simulink model "Simulator_Case_5"  (R2024a)
settings: Solver=VariableStepAuto  StartTime=0.0  StopTime=2800  RelTol=1e-3
values from neighbouring files (symbols this model uses):
  Heading_Initial = -65*pi/180    (= -1.1344640138)    [Parametrization_Simulation_Case_5.m]
  Position_Initial_X = Waypoints_X(1)    [Parametrization_Simulation_Case_5.m]
  Position_Initial_Y = Waypoints_Y(1)    [Parametrization_Simulation_Case_5.m]
  Time_Period_Sampling = 0.1    [Parametrization_Simulation_Case_5.m]
undefined symbols (not defined in the file or in its folder): Area_Lateral_Projected_Wind, Damping_Factor_Waves, Density_Air, DiscIntNeverNeededParam, Gain_Proportional, Inertia_Moment, Length_Ship, Pulsation_Wave, Rudder_To_Heading_Discretized, Static_Gain_Nomoto, Structure_Wind_Coefficient, Time_Constant_Total, Time_Derivative, Time_Integral, Velocity_Ship_Mean, Wave_Transfer_Function_Discrete, Waypoints, Yaw_Control_Hydrodynamics_Derivative
libraries: simulink_extras x4, sensorgpslib x1
settings Model: Creator=gerar  LastModifiedBy=gerar

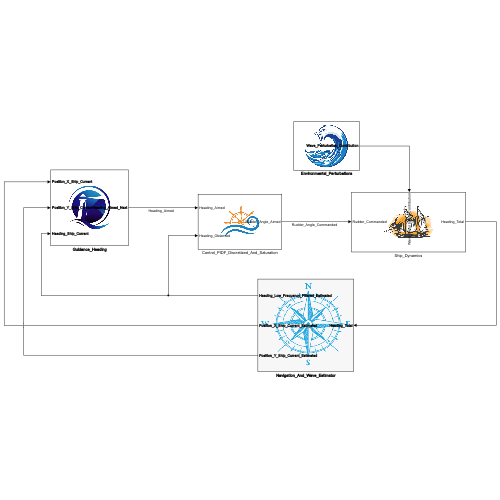
[thumbnail: Simulink's stored preview of the top-level diagram]
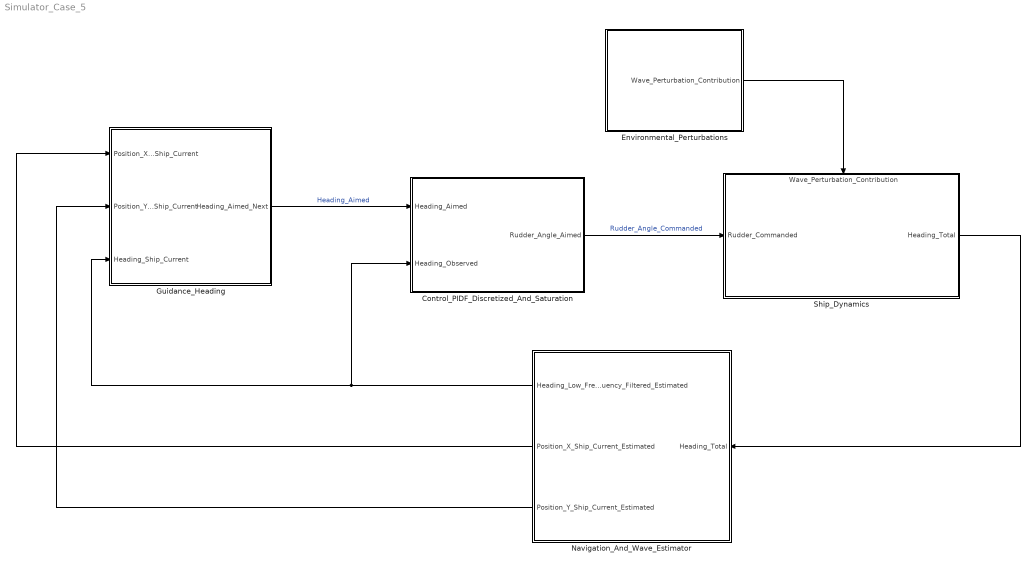
== system Simulator_Case_5 ==
  Control_PIDF_Discretized_And_Saturation : Subsystem
      mask Display: image('Rudder3.jpg');
  Environmental_Perturbations : Subsystem
      mask Display: image('Wave2.png');
  Guidance_Heading : Subsystem
      mask Display: image('phare4.jpg');
  Navigation_And_Wave_Estimator : Subsystem
      mask Display: image('compass4.png');
  Ship_Dynamics : Subsystem
      settings: PortSchema="{\"entries\":[{\"content\":{\"sides\":[{\"content\":{\"connectorIds\":[\"In1\"]},\"type\":\"ConnectorPlacement.EquallySpacedRectSide\",\"uuid\":\"1262d93f-9737-49c5-b1c8-13d3f825160d\"},{\"content\":{\"connectorIds\":[\"Out1\"],\"side\":\"RIGHT\"},\"type\":\"ConnectorPlacement.EquallySpacedRectSide\",\"uuid\":\"2783823e-17f0-4da0-9b4a-e84aa912eb5f\"},{\"content\":{\"connectorIds\":[\"In2\"],\"side\":\"TOP\"},\"type\":\"ConnectorPlacement.EquallySpacedRectSide\",\"uuid\":\"9227960a-c500-4bd1-9392-f2e1de824969\"}]},\"type\":\"ConnectorPlacement.EquallySpacedConnector\",\"uuid\":\"fe1a7a14-057d-49da-982c-994c0d128614\"}],\"packageUris\":[\"http://schema.mathworks.com/mf0/Connector/R2020b\"],\"version\":\"1.0\"}"
      mask Display: image('ship2.png');
  wires:
  Guidance_Heading/1(Heading_Aimed_Next) -> Control_PIDF_Discretized_And_Saturation/1(Heading_Aimed)  "Heading_Aimed"
  Navigation_And_Wave_Estimator/1(Heading_Low_Frequency_Filtered_Estimated) -> Control_PIDF_Discretized_And_Saturation/2(Heading_Observed), Guidance_Heading/3(Heading_Ship_Current)
  Control_PIDF_Discretized_And_Saturation/1(Rudder_Angle_Aimed) -> Ship_Dynamics/1(Rudder_Commanded)  "Rudder_Angle_Commanded"
  Environmental_Perturbations/1(Wave_Perturbation_Contribution) -> Ship_Dynamics/2(Wave_Perturbation_Contribution)
  Ship_Dynamics/1(Heading_Total) -> Navigation_And_Wave_Estimator/1(Heading_Total)
  Navigation_And_Wave_Estimator/3(Position_Y_Ship_Current_Estimated) -> Guidance_Heading/2(Position_Y_Ship_Current)
  Navigation_And_Wave_Estimator/2(Position_X_Ship_Current_Estimated) -> Guidance_Heading/1(Position_X_Ship_Current)

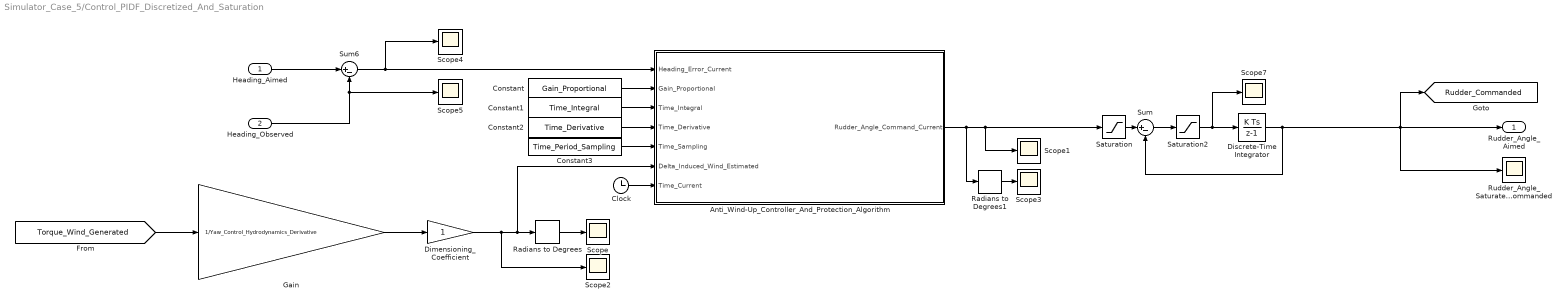
== system Simulator_Case_5/Control_PIDF_Discretized_And_Saturation ==
  Heading_Aimed : Inport
  Heading_Observed : Inport  Port=2
  Anti_Wind-Up_Controller_And_Protection_Algorithm : MATLAB Function  TreatAsAtomicUnit=on  SystemSampleTime=Time_Period_Sampling
  Clock : Clock
  Constant : Constant  Value=Gain_Proportional
  Constant1 : Constant  Value=Time_Integral
  Constant2 : Constant  Value=Time_Derivative
  Constant3 : Constant  Value=Time_Period_Sampling
  Dimensioning_Coefficient : Gain
  Discrete-Time Integrator : DiscreteIntegrator  SampleTime=Time_Period_Sampling  ICPrevOutput=DiscIntNeverNeededParam  ICPrevScaledInput=DiscIntNeverNeededParam
  Gain : Gain  Gain=1/Yaw_Control_Hydrodynamics_Derivative
  Radians to Degrees : simulink_extras/Transformations/Radians to Degrees
  Radians to Degrees1 : simulink_extras/Transformations/Radians to Degrees
  Rudder_Angle_Saturated_Commanded : Scope
  Saturation : Saturate  UpperLimit=35*(pi/180)  LowerLimit=-35*(pi/180)
  Saturation2 : Saturate  UpperLimit=15*(pi/180)  LowerLimit=-15*(pi/180)
  Scope{,1..5,7} (7 alike) : Scope
  Sum : Sum  Inputs=|+-
  Sum6 : Sum  Inputs=|+-
  Rudder_Angle_Aimed : Outport
  tag scope: Rudder_Commanded=global
  wires:
  Sum6/1 -> Scope4/1, Anti_Wind-Up_Controller_And_Protection_Algorithm/1(Heading_Error_Current)
  Heading_Aimed/1 -> Sum6/1
  Heading_Observed/1 -> Scope5/1, Sum6/2
  Constant/1 -> Anti_Wind-Up_Controller_And_Protection_Algorithm/2(Gain_Proportional)
  Constant1/1 -> Anti_Wind-Up_Controller_And_Protection_Algorithm/3(Time_Integral)
  Constant2/1 -> Anti_Wind-Up_Controller_And_Protection_Algorithm/4(Time_Derivative)
  Constant3/1 -> Anti_Wind-Up_Controller_And_Protection_Algorithm/5(Time_Sampling)
  [Torque_Wind_Generated] -> Gain/1
  Gain/1 -> Dimensioning_Coefficient/1
  Radians to Degrees/1 -> Scope/1
  Radians to Degrees1/1 -> Scope3/1
  Anti_Wind-Up_Controller_And_Protection_Algorithm/1(Rudder_Angle_Command_Current) -> Radians to Degrees1/1, Saturation/1, Scope1/1
  Dimensioning_Coefficient/1 -> Anti_Wind-Up_Controller_And_Protection_Algorithm/6(Delta_Induced_Wind_Estimated), Radians to Degrees/1, Scope2/1
  Clock/1 -> Anti_Wind-Up_Controller_And_Protection_Algorithm/7(Time_Current)
  Saturation2/1 -> Scope7/1, Discrete-Time Integrator/1
  Saturation/1 -> Sum/1
  Sum/1 -> Saturation2/1
  Discrete-Time Integrator/1 -> Sum/2, Rudder_Angle_Saturated_Commanded/1, [Rudder_Commanded], Rudder_Angle_Aimed/1

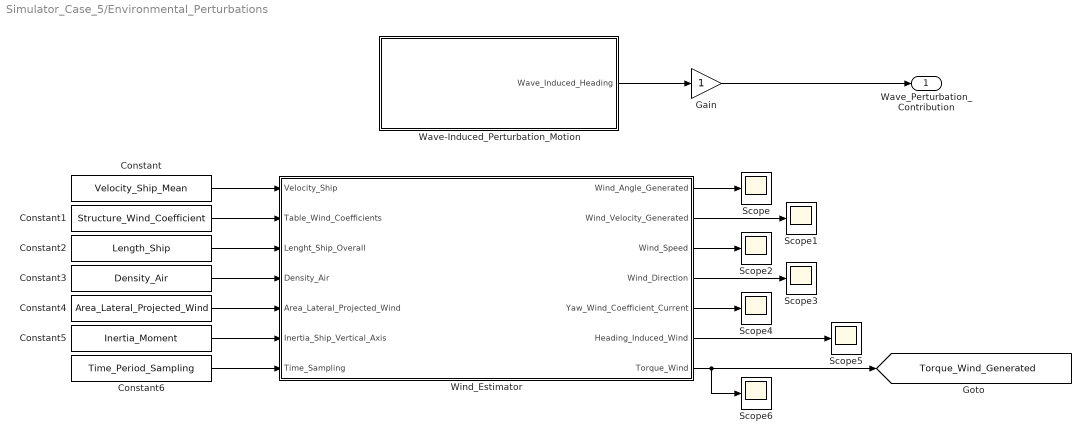
== system Simulator_Case_5/Environmental_Perturbations ==
  Constant : Constant  Value=Velocity_Ship_Mean
  Constant1 : Constant  Value=Structure_Wind_Coefficient
  Constant2 : Constant  Value=Length_Ship
  Constant3 : Constant  Value=Density_Air
  Constant4 : Constant  Value=Area_Lateral_Projected_Wind
  Constant5 : Constant  Value=Inertia_Moment
  Constant6 : Constant  Value=Time_Period_Sampling
  Gain : Gain
  Scope{,1..6} (7 alike) : Scope
  Wave-Induced_Perturbation_Motion : Subsystem
  Wind_Estimator : MATLAB Function  TreatAsAtomicUnit=on  SystemSampleTime=Time_Period_Sampling
  Wave_Perturbation_Contribution : Outport
  tag scope: Torque_Wind_Generated=global
  wires:
  Wave-Induced_Perturbation_Motion/1(Wave_Induced_Heading) -> Gain/1
  Constant/1 -> Wind_Estimator/1(Velocity_Ship)
  Constant1/1 -> Wind_Estimator/2(Table_Wind_Coefficients)
  Constant2/1 -> Wind_Estimator/3(Lenght_Ship_Overall)
  Constant3/1 -> Wind_Estimator/4(Density_Air)
  Constant4/1 -> Wind_Estimator/5(Area_Lateral_Projected_Wind)
  Constant5/1 -> Wind_Estimator/6(Inertia_Ship_Vertical_Axis)
  Wind_Estimator/1(Wind_Angle_Generated) -> Scope/1
  Wind_Estimator/2(Wind_Velocity_Generated) -> Scope1/1
  Wind_Estimator/3(Wind_Speed) -> Scope2/1
  Wind_Estimator/4(Wind_Direction) -> Scope3/1
  Wind_Estimator/5(Yaw_Wind_Coefficient_Current) -> Scope4/1
  Wind_Estimator/6(Heading_Induced_Wind) -> Scope5/1
  Wind_Estimator/7(Torque_Wind) -> Scope6/1, [Torque_Wind_Generated]
  Constant6/1 -> Wind_Estimator/7(Time_Sampling)
  Gain/1 -> Wave_Perturbation_Contribution/1

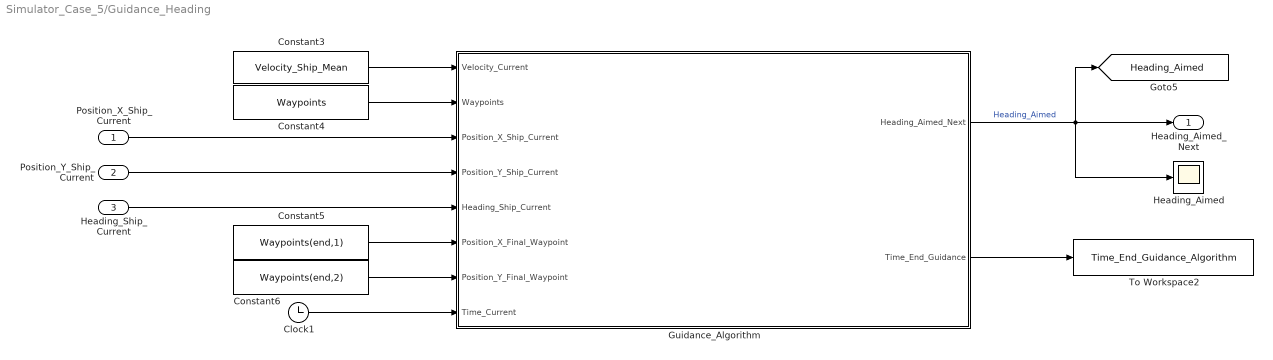
== system Simulator_Case_5/Guidance_Heading ==
  Position_X_Ship_Current : Inport
  Position_Y_Ship_Current : Inport  Port=2
  Heading_Ship_Current : Inport  Port=3
  Clock1 : Clock
  Constant3 : Constant  Value=Velocity_Ship_Mean
  Constant4 : Constant  Value=Waypoints
  Constant5 : Constant  Value=Waypoints(end,1)
  Constant6 : Constant  Value=Waypoints(end,2)
  Guidance_Algorithm : MATLAB Function  TreatAsAtomicUnit=on  SystemSampleTime=20
  Heading_Aimed : Scope
  To Workspace2 : ToWorkspace  VariableName=Time_End_Guidance_Algorithm  SaveFormat=Timeseries  SampleTime=-1
  Heading_Aimed_Next : Outport
  tag scope: Heading_Aimed=global
  wires:
  Constant5/1 -> Guidance_Algorithm/6(Position_X_Final_Waypoint)
  Guidance_Algorithm/2(Time_End_Guidance) -> To Workspace2/1
  Constant3/1 -> Guidance_Algorithm/1(Velocity_Current)
  Position_Y_Ship_Current/1 -> Guidance_Algorithm/4(Position_Y_Ship_Current)
  Constant4/1 -> Guidance_Algorithm/2(Waypoints)
  Clock1/1 -> Guidance_Algorithm/8(Time_Current)
  Constant6/1 -> Guidance_Algorithm/7(Position_Y_Final_Waypoint)
  Position_X_Ship_Current/1 -> Guidance_Algorithm/3(Position_X_Ship_Current)
  Heading_Ship_Current/1 -> Guidance_Algorithm/5(Heading_Ship_Current)
  Guidance_Algorithm/1(Heading_Aimed_Next) -> Heading_Aimed/1, Heading_Aimed_Next/1, [Heading_Aimed]  "Heading_Aimed"

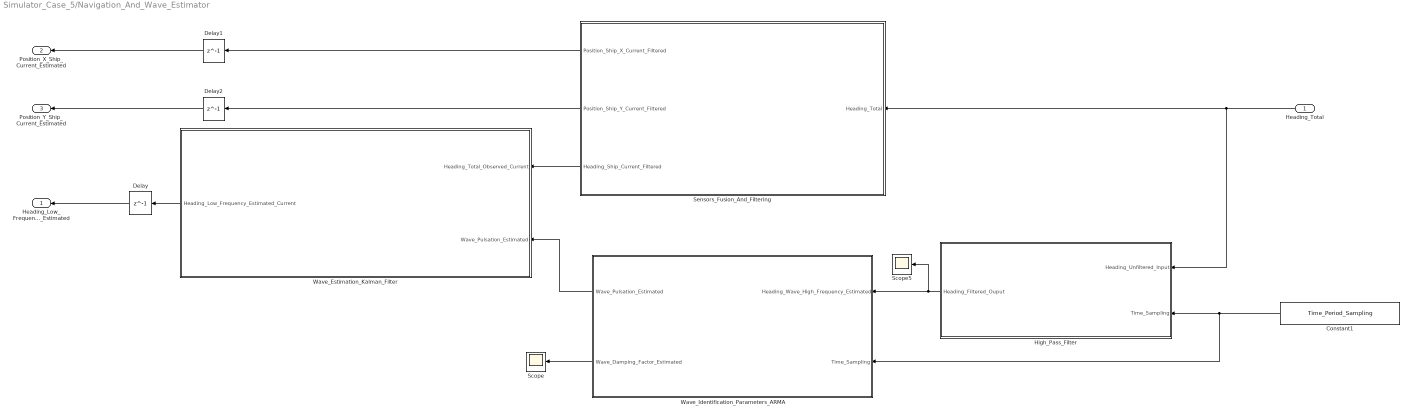
== system Simulator_Case_5/Navigation_And_Wave_Estimator ==
  Heading_Total : Inport
  Constant1 : Constant  Value=Time_Period_Sampling
  Delay : Delay  DelayLength=1  InputProcessing=Columns as channels (frame based)  SampleTime=0.1
  Delay1 : Delay  DelayLength=1  InputProcessing=Columns as channels (frame based)  SampleTime=0.1
  Delay2 : Delay  DelayLength=1  InputProcessing=Columns as channels (frame based)  SampleTime=0.1
  High_Pass_Filter : MATLAB Function  TreatAsAtomicUnit=on  SystemSampleTime=Time_Period_Sampling
  Scope : Scope
  Scope5 : Scope
  Sensors_Fusion_And_Filtering : Subsystem
  Wave_Estimation_Kalman_Filter : Subsystem
  Wave_Identification_Parameters_ARMA : MATLAB Function  TreatAsAtomicUnit=on  SystemSampleTime=Time_Period_Sampling
  Heading_Low_Frequency_Filtered_Estimated : Outport
  Position_X_Ship_Current_Estimated : Outport  Port=2
  Position_Y_Ship_Current_Estimated : Outport  Port=3
  wires:
  Delay/1 -> Heading_Low_Frequency_Filtered_Estimated/1
  Delay1/1 -> Position_X_Ship_Current_Estimated/1
  Delay2/1 -> Position_Y_Ship_Current_Estimated/1
  Sensors_Fusion_And_Filtering/1(Position_Ship_X_Current_Filtered) -> Delay1/1
  Sensors_Fusion_And_Filtering/2(Position_Ship_Y_Current_Filtered) -> Delay2/1
  Sensors_Fusion_And_Filtering/3(Heading_Ship_Current_Filtered) -> Wave_Estimation_Kalman_Filter/1(Heading_Total_Observed_Current)
  Wave_Estimation_Kalman_Filter/1(Heading_Low_Frequency_Estimated_Current) -> Delay/1
  High_Pass_Filter/1(Heading_Filtered_Ouput) -> Scope5/1, Wave_Identification_Parameters_ARMA/1(Heading_Wave_High_Frequency_Estimated)
  Constant1/1 -> Wave_Identification_Parameters_ARMA/2(Time_Sampling), High_Pass_Filter/2(Time_Sampling)
  Wave_Identification_Parameters_ARMA/2(Wave_Damping_Factor_Estimated) -> Scope/1
  Wave_Identification_Parameters_ARMA/1(Wave_Pulsation_Estimated) -> Wave_Estimation_Kalman_Filter/2(Wave_Pulsation_Estimated)
  Heading_Total/1 -> High_Pass_Filter/1(Heading_Unfiltered_Input), Sensors_Fusion_And_Filtering/1(Heading_Total)

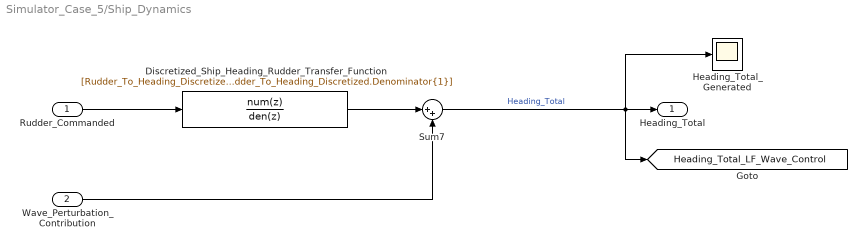
== system Simulator_Case_5/Ship_Dynamics ==
  Rudder_Commanded : Inport
  Wave_Perturbation_Contribution : Inport  Port=2
  Discretized_Ship_Heading_Rudder_Transfer_Function : DiscreteTransferFcn  Numerator=[Rudder_To_Heading_Discretized.Numerator{1}]  Denominator=[Rudder_To_Heading_Discretized.Denominator{1}]  InitialStates=Heading_Initial
  Heading_Total_Generated : Scope
  Sum7 : Sum  Inputs=|++
  Heading_Total : Outport
  tag scope: Heading_Total_LF_Wave_Control=global
  wires:
  Discretized_Ship_Heading_Rudder_Transfer_Function/1 -> Sum7/1
  Wave_Perturbation_Contribution/1 -> Sum7/2
  Rudder_Commanded/1 -> Discretized_Ship_Heading_Rudder_Transfer_Function/1
  Sum7/1 -> [Heading_Total_LF_Wave_Control], Heading_Total/1, Heading_Total_Generated/1  "Heading_Total"

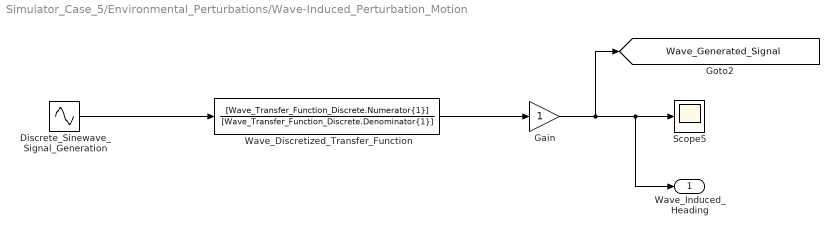
== system Simulator_Case_5/Environmental_Perturbations/Wave-Induced_Perturbation_Motion ==
  Discrete_Sinewave_Signal_Generation : Sin  Amplitude=5*(pi/180)  Frequency=Pulsation_Wave  SampleTime=Time_Period_Sampling
  Gain : Gain
  Scope5 : Scope
  Wave_Discretized_Transfer_Function : DiscreteTransferFcn  Numerator=[Wave_Transfer_Function_Discrete.Numerator{1}]  Denominator=[Wave_Transfer_Function_Discrete.Denominator{1}]
  Wave_Induced_Heading : Outport
  tag scope: Wave_Generated_Signal=global
  wires:
  Gain/1 -> Wave_Induced_Heading/1, Scope5/1, [Wave_Generated_Signal]
  Discrete_Sinewave_Signal_Generation/1 -> Wave_Discretized_Transfer_Function/1
  Wave_Discretized_Transfer_Function/1 -> Gain/1

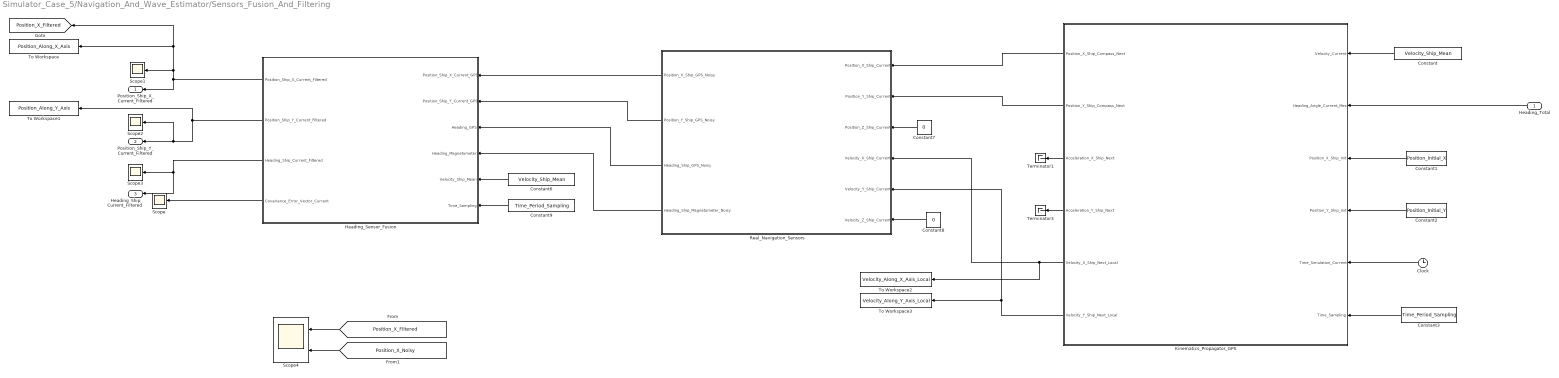
== system Simulator_Case_5/Navigation_And_Wave_Estimator/Sensors_Fusion_And_Filtering ==
  Heading_Total : Inport
  Clock : Clock
  Constant : Constant  Value=Velocity_Ship_Mean
  Constant1 : Constant  Value=Position_Initial_X
  Constant2 : Constant  Value=Position_Initial_Y
  Constant3 : Constant  Value=Time_Period_Sampling
  Constant6 : Constant  Value=Velocity_Ship_Mean
  Constant7 : Constant  Value=0
  Constant8 : Constant  Value=0
  Constant9 : Constant  Value=Time_Period_Sampling
  Heading_Sensor_Fusion : MATLAB Function  TreatAsAtomicUnit=on  SystemSampleTime=Time_Period_Sampling
  Kinematics_Propagator_GPS : MATLAB Function  TreatAsAtomicUnit=on  SystemSampleTime=Time_Period_Sampling
  Real_Navigation_Sensors : Subsystem
  Scope{,1..3} (4 alike) : Scope
  Scope4 : Scope  NumInputPorts=2
  Terminator1 : Terminator
  Terminator3 : Terminator
  To Workspace : ToWorkspace  VariableName=Position_Along_X_Axis  SaveFormat=Timeseries  SampleTime=Time_Period_Sampling
  To Workspace1 : ToWorkspace  VariableName=Position_Along_Y_Axis  SaveFormat=Timeseries  SampleTime=Time_Period_Sampling
  To Workspace2 : ToWorkspace  VariableName=Velocity_Along_X_Axis_Local  SaveFormat=Timeseries  SampleTime=Time_Period_Sampling
  To Workspace3 : ToWorkspace  VariableName=Velocity_Along_Y_Axis_Local  SaveFormat=Timeseries  SampleTime=Time_Period_Sampling
  Position_Ship_X_Current_Filtered : Outport
  Position_Ship_Y_Current_Filtered : Outport  Port=2
  Heading_Ship_Current_Filtered : Outport  Port=3
  tag scope: Position_X_Filtered=global
  wires:
  Real_Navigation_Sensors/1(Position_X_Ship_GPS_Noisy) -> Heading_Sensor_Fusion/1(Position_Ship_X_Current_GPS)
  Real_Navigation_Sensors/3(Heading_Ship_GPS_Noisy) -> Heading_Sensor_Fusion/3(Heading_GPS)
  Constant6/1 -> Heading_Sensor_Fusion/5(Velocity_Ship_Mean)
  Real_Navigation_Sensors/4(Heading_Ship_Magnetometer_Noisy) -> Heading_Sensor_Fusion/4(Heading_Magnetometer)
  Real_Navigation_Sensors/2(Position_Y_Ship_GPS_Noisy) -> Heading_Sensor_Fusion/2(Position_Ship_Y_Current_GPS)
  Constant2/1 -> Kinematics_Propagator_GPS/4(Position_Y_Ship_Init)
  Heading_Total/1 -> Kinematics_Propagator_GPS/2(Heading_Angle_Current_Mes)
  Clock/1 -> Kinematics_Propagator_GPS/5(Time_Simulation_Current)
  Constant1/1 -> Kinematics_Propagator_GPS/3(Position_X_Ship_Init)
  Constant/1 -> Kinematics_Propagator_GPS/1(Velocity_Current)
  Constant3/1 -> Kinematics_Propagator_GPS/6(Time_Sampling)
  Kinematics_Propagator_GPS/1(Position_X_Ship_Compass_Next) -> Real_Navigation_Sensors/1(Position_X_Ship_Current)
  Kinematics_Propagator_GPS/2(Position_Y_Ship_Compass_Next) -> Real_Navigation_Sensors/2(Position_Y_Ship_Current)
  Kinematics_Propagator_GPS/5(Velocity_X_Ship_Next_Local) -> Real_Navigation_Sensors/4(Velocity_X_Ship_Current), To Workspace2/1
  Kinematics_Propagator_GPS/6(Velocity_Y_Ship_Next_Local) -> To Workspace3/1, Real_Navigation_Sensors/5(Velocity_Y_Ship_Current)
  Constant7/1 -> Real_Navigation_Sensors/3(Position_Z_Ship_Current)
  Constant8/1 -> Real_Navigation_Sensors/6(Velocity_Z_Ship_Current)
  Constant9/1 -> Heading_Sensor_Fusion/6(Time_Sampling)
  Heading_Sensor_Fusion/1(Position_Ship_X_Current_Filtered) -> Position_Ship_X_Current_Filtered/1, [Position_X_Filtered], To Workspace/1, Scope1/1
  Heading_Sensor_Fusion/2(Position_Ship_Y_Current_Filtered) -> Scope2/1, Position_Ship_Y_Current_Filtered/1, To Workspace1/1
  Heading_Sensor_Fusion/3(Heading_Ship_Current_Filtered) -> Heading_Ship_Current_Filtered/1, Scope3/1
  Heading_Sensor_Fusion/4(Covariance_Error_Vector_Current) -> Scope/1
  Kinematics_Propagator_GPS/3(Acceleration_X_Ship_Next) -> Terminator1/1
  Kinematics_Propagator_GPS/4(Acceleration_Y_Ship_Next) -> Terminator3/1
  [Position_X_Filtered] -> Scope4/1
  [Position_X_Noisy] -> Scope4/2

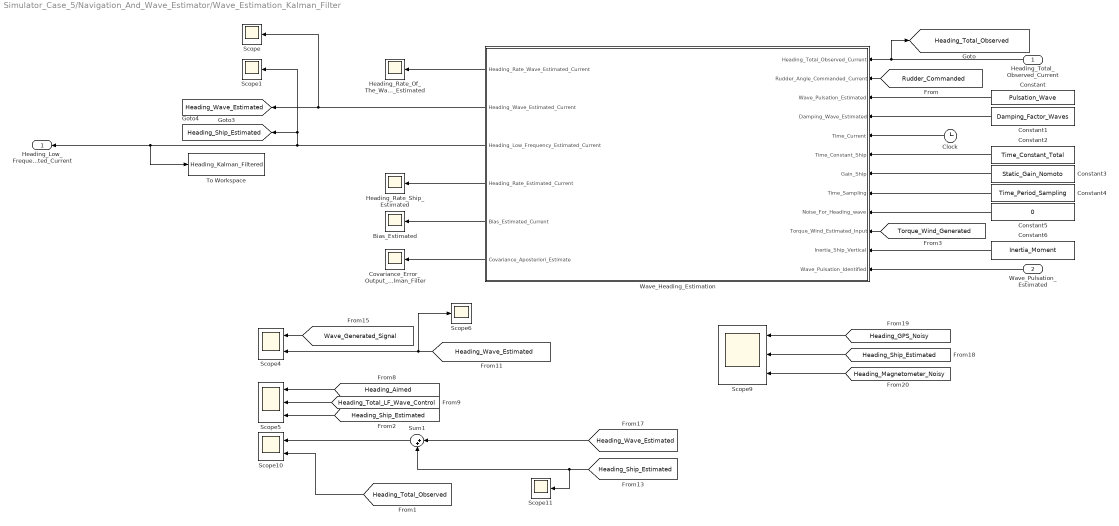
== system Simulator_Case_5/Navigation_And_Wave_Estimator/Wave_Estimation_Kalman_Filter ==
  Heading_Total_Observed_Current : Inport
  Wave_Pulsation_Estimated : Inport  Port=2
  Bias_Estimated : Scope
  Clock : Clock
  Constant : Constant  Value=Pulsation_Wave  SampleTime=Time_Period_Sampling
  Constant1 : Constant  Value=Damping_Factor_Waves  SampleTime=Time_Period_Sampling
  Constant2 : Constant  Value=Time_Constant_Total  SampleTime=Time_Period_Sampling
  Constant3 : Constant  Value=Static_Gain_Nomoto  SampleTime=Time_Period_Sampling
  Constant4 : Constant  Value=Time_Period_Sampling  SampleTime=Time_Period_Sampling
  Constant5 : Constant  Value=0
  Constant6 : Constant  Value=Inertia_Moment
  Covariance_Error_Output_Kalman_Filter : Scope
  Heading_Rate_Of_The_Waves_Estimated : Scope
  Heading_Rate_Ship_Estimated : Scope
  Scope{,1,6,11} (4 alike) : Scope
  Scope10 : Scope  NumInputPorts=2
  Scope4 : Scope  NumInputPorts=2
  Scope5 : Scope  NumInputPorts=3
  Scope9 : Scope  NumInputPorts=3
  Sum1 : Sum  Inputs=|++
  To Workspace : ToWorkspace  VariableName=Heading_Kalman_Filtered  SaveFormat=Timeseries  SampleTime=Time_Period_Sampling
  Wave_Heading_Estimation : MATLAB Function  TreatAsAtomicUnit=on  SystemSampleTime=Time_Period_Sampling
  Heading_Low_Frequency_Estimated_Current : Outport
  tag scope: Heading_Ship_Estimated=global, Heading_Total_Observed=global, Heading_Wave_Estimated=global
  wires:
  Wave_Heading_Estimation/3(Heading_Low_Frequency_Estimated_Current) -> Scope1/1, [Heading_Ship_Estimated], Heading_Low_Frequency_Estimated_Current/1, To Workspace/1
  Heading_Total_Observed_Current/1 -> [Heading_Total_Observed], Wave_Heading_Estimation/1(Heading_Total_Observed_Current)
  [Rudder_Commanded] -> Wave_Heading_Estimation/2(Rudder_Angle_Commanded_Current)
  Constant/1 -> Wave_Heading_Estimation/3(Wave_Pulsation_Estimated)
  Constant1/1 -> Wave_Heading_Estimation/4(Damping_Wave_Estimated)
  Clock/1 -> Wave_Heading_Estimation/5(Time_Current)
  Constant2/1 -> Wave_Heading_Estimation/6(Time_Constant_Ship)
  Constant3/1 -> Wave_Heading_Estimation/7(Gain_Ship)
  Constant4/1 -> Wave_Heading_Estimation/8(Time_Sampling)
  Constant5/1 -> Wave_Heading_Estimation/9(Noise_For_Heading_wave)
  Wave_Heading_Estimation/1(Heading_Rate_Wave_Estimated_Current) -> Heading_Rate_Of_The_Waves_Estimated/1
  Wave_Heading_Estimation/2(Heading_Wave_Estimated_Current) -> Scope/1, [Heading_Wave_Estimated]
  Wave_Heading_Estimation/5(Bias_Estimated_Current) -> Bias_Estimated/1
  Wave_Heading_Estimation/4(Heading_Rate_Estimated_Current) -> Heading_Rate_Ship_Estimated/1
  Wave_Heading_Estimation/6(Covariance_Aposteriori_Estimate) -> Covariance_Error_Output_Kalman_Filter/1
  [Heading_Aimed] -> Scope5/1
  [Wave_Generated_Signal] -> Scope4/1
  [Heading_Ship_Estimated] -> Scope9/2
  [Heading_Magnetometer_Noisy] -> Scope9/3
  [Heading_Ship_Estimated] -> Scope11/1, Sum1/2
  [Heading_GPS_Noisy] -> Scope9/1
  [Heading_Wave_Estimated] -> Sum1/1
  Sum1/1 -> Scope10/1
  [Heading_Total_LF_Wave_Control] -> Scope5/2
  [Heading_Ship_Estimated] -> Scope5/3
  [Heading_Wave_Estimated] -> Scope6/1, Scope4/2
  [Heading_Total_Observed] -> Scope10/2
  Constant6/1 -> Wave_Heading_Estimation/11(Inertia_Ship_Vertical)
  [Torque_Wind_Generated] -> Wave_Heading_Estimation/10(Torque_Wind_Estimated_Input)
  Wave_Pulsation_Estimated/1 -> Wave_Heading_Estimation/12(Wave_Pulsation_Identified)

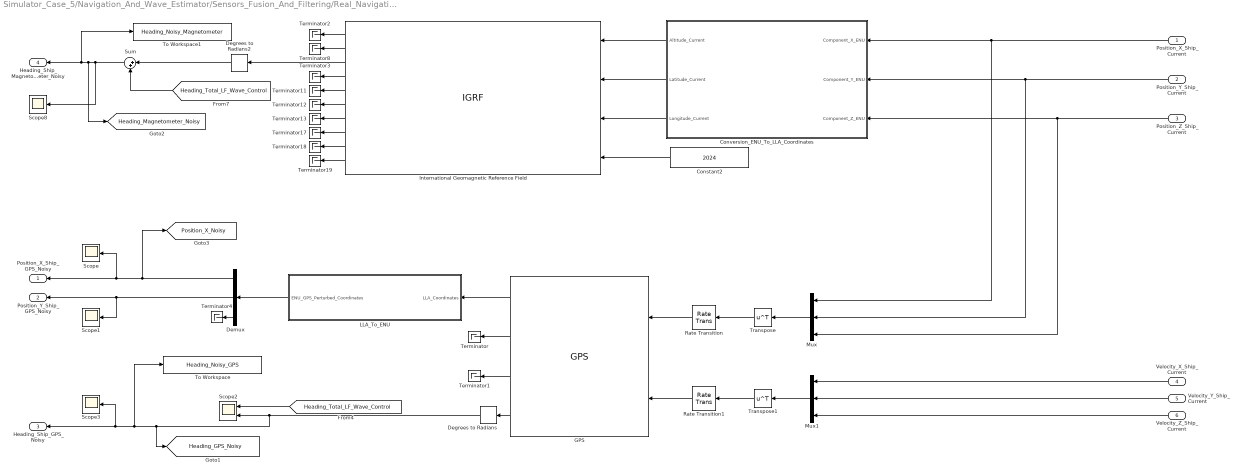
== system Simulator_Case_5/Navigation_And_Wave_Estimator/Sensors_Fusion_And_Filtering/Real_Navigation_Sensors ==
  Position_X_Ship_Current : Inport
  Position_Y_Ship_Current : Inport  Port=2
  Position_Z_Ship_Current : Inport  Port=3
  Velocity_X_Ship_Current : Inport  Port=4
  Velocity_Y_Ship_Current : Inport  Port=5
  Velocity_Z_Ship_Current : Inport  Port=6
  Constant2 : Constant  Value=2024
  Conversion_ENU_To_LLA_Coordinates : MATLAB Function  TreatAsAtomicUnit=on  SystemSampleTime=Time_Period_Sampling
  Degrees to Radians : simulink_extras/Transformations/Degrees to Radians
  Degrees to Radians2 : simulink_extras/Transformations/Degrees to Radians
  Demux : Demux  Outputs=3
  GPS : sensorgpslib/GPS  DispRefFrame=ENU  PositionInputFormat=Local  ReferenceLocation=[43.059023, 3.002915 ,0]  HorizontalPositionAccuracy=2  VerticalPositionAccuracy=2  VelocityAccuracy=0.1  DecayFactor=0.999  SeedDouble=67  SimulateUsing=Interpreted execution
  International Geomagnetic Reference Field : IGRF  month=January  day=1  year=2020
      settings: AttributesFormatString=%<generation>
  LLA_To_ENU : MATLAB Function  TreatAsAtomicUnit=on  SystemSampleTime=Time_Period_Sampling
  Mux : Mux  Inputs=3
  Mux1 : Mux  Inputs=3
  Rate Transition : RateTransition  OutPortSampleTime=Time_Period_Sampling
  Rate Transition1 : RateTransition  OutPortSampleTime=Time_Period_Sampling
  Scope{,1,3,8} (4 alike) : Scope
  Scope2 : Scope  NumInputPorts=2
  Sum : Sum  Inputs=|++
  Terminator{,1..4,8,11..13,17..19} (12 alike) : Terminator
  To Workspace : ToWorkspace  VariableName=Heading_Noisy_GPS  SaveFormat=Timeseries  SampleTime=Time_Period_Sampling
  To Workspace1 : ToWorkspace  VariableName=Heading_Noisy_Magnetometer  SaveFormat=Timeseries  SampleTime=Time_Period_Sampling
  Transpose : Math  Operator=transpose
  Transpose1 : Math  Operator=transpose
  Position_X_Ship_GPS_Noisy : Outport
  Position_Y_Ship_GPS_Noisy : Outport  Port=2
  Heading_Ship_GPS_Noisy : Outport  Port=3
  Heading_Ship_Magnetometer_Noisy : Outport  Port=4
  tag scope: Heading_GPS_Noisy=global, Heading_Magnetometer_Noisy=global, Position_X_Noisy=global
  wires:
  [Heading_Total_LF_Wave_Control] -> Scope2/1
  International Geomagnetic Reference Field/1 -> Terminator2/1
  Position_Y_Ship_Current/1 -> Mux/2, Conversion_ENU_To_LLA_Coordinates/2(Component_Y_ENU)
  GPS/3 -> Terminator1/1
  International Geomagnetic Reference Field/6 -> Terminator12/1
  International Geomagnetic Reference Field/10 -> Terminator19/1
  Demux/2 -> Position_Y_Ship_GPS_Noisy/1, Scope1/1
  International Geomagnetic Reference Field/5 -> Terminator11/1
  Degrees to Radians/1 -> [Heading_GPS_Noisy], To Workspace/1, Heading_Ship_GPS_Noisy/1, Scope3/1, Scope2/2
  Velocity_Y_Ship_Current/1 -> Mux1/2
  Conversion_ENU_To_LLA_Coordinates/1(Altitude_Current) -> International Geomagnetic Reference Field/1
  Demux/3 -> Terminator4/1
  Degrees to Radians2/1 -> Sum/1
  Mux/1 -> Transpose/1
  Position_X_Ship_Current/1 -> Mux/1, Conversion_ENU_To_LLA_Coordinates/1(Component_X_ENU)
  [Heading_Total_LF_Wave_Control] -> Sum/2
  Constant2/1 -> International Geomagnetic Reference Field/4
  GPS/4 -> Degrees to Radians/1
  GPS/2 -> Terminator/1
  International Geomagnetic Reference Field/4 -> Terminator3/1
  Rate Transition1/1 -> GPS/2
  Demux/1 -> [Position_X_Noisy], Position_X_Ship_GPS_Noisy/1, Scope/1
  International Geomagnetic Reference Field/8 -> Terminator17/1
  International Geomagnetic Reference Field/2 -> Terminator8/1
  Transpose1/1 -> Rate Transition1/1
  Conversion_ENU_To_LLA_Coordinates/2(Latitude_Current) -> International Geomagnetic Reference Field/2
  Transpose/1 -> Rate Transition/1
  Rate Transition/1 -> GPS/1
  Position_Z_Ship_Current/1 -> Mux/3, Conversion_ENU_To_LLA_Coordinates/3(Component_Z_ENU)
  LLA_To_ENU/1(ENU_GPS_Perturbed_Coordinates) -> Demux/1
  Mux1/1 -> Transpose1/1
  International Geomagnetic Reference Field/3 -> Degrees to Radians2/1
  GPS/1 -> LLA_To_ENU/1(LLA_Coordinates)
  Conversion_ENU_To_LLA_Coordinates/3(Longitude_Current) -> International Geomagnetic Reference Field/3
  International Geomagnetic Reference Field/7 -> Terminator13/1
  International Geomagnetic Reference Field/9 -> Terminator18/1
  Velocity_Z_Ship_Current/1 -> Mux1/3
  Velocity_X_Ship_Current/1 -> Mux1/1
  Sum/1 -> To Workspace1/1, Heading_Ship_Magnetometer_Noisy/1, [Heading_Magnetometer_Noisy], Scope8/1

== matlab function Simulator_Case_5/Navigation_And_Wave_Estimator/Sensors_Fusion_And_Filtering/Heading_Sensor_Fusion ==
  settings: updateMethod=DISCRETE
  data: Position_Ship_X_Current_GPS input; Position_Ship_Y_Current_GPS input; Heading_GPS input; Heading_Magnetometer input; Position_Ship_X_Current_Filtered output; Position_Ship_Y_Current_Filtered output; Heading_Ship_Current_Filtered output; Covariance_Error_Vector_Current output; Velocity_Ship_Mean input; Time_Sampling input
function [Position_Ship_X_Current_Filtered,...
          Position_Ship_Y_Current_Filtered,...
          Heading_Ship_Current_Filtered,...
          Covariance_Error_Vector_Current]  = Navigation_Kalman_Sensor_Fusion(Position_Ship_X_Current_GPS,...
                                                                              Position_Ship_Y_Current_GPS,...
                                                                              Heading_GPS,...
                                                                              Heading_Magnetometer,...
                                                                              Velocity_Ship_Mean,...
                                                                              Time_Sampling)

% Online Sensor Fusion and Filtering algorithm:
[Position_Ship_X_Current_Filtered,...
 Position_Ship_Y_Current_Filtered,...
 Heading_Ship_Current_Filtered,...
 Covariance_Error_Vector_Current] = Navigation_Kalman_Fusion_Positions_Heading(Position_Ship_X_Current_GPS,...
                                                                               Position_Ship_Y_Current_GPS,...
                                                                               Heading_GPS,...
                                                                               Heading_Magnetometer,...
                                                                               Velocity_Ship_Mean,...
                                                                               Time_Sampling);

end

== matlab function Simulator_Case_5/Navigation_And_Wave_Estimator/Sensors_Fusion_And_Filtering/Real_Navigation_Sensors/LLA_To_ENU ==
  data: LLA_Coordinates input; ENU_GPS_Perturbed_Coordinates output
function ENU_GPS_Perturbed_Coordinates = Conversion_LLA_To_ENU(LLA_Coordinates)

% Reference point:
Reference_Point_Port_Mahon = [43.059023,3.002915,0];
Semi_Major_Axis = 6378137.0;
Flattening = 1/298.25;

% This function serves as a mean to convert LLA coordinates to ENU
% coordinates:
ENU_GPS_Perturbed_Coordinates = LLA_To_ENU(LLA_Coordinates(1),LLA_Coordinates(2),LLA_Coordinates(3),...
                                           Reference_Point_Port_Mahon(1),Reference_Point_Port_Mahon(2),...
                                           Reference_Point_Port_Mahon(3),Semi_Major_Axis,Flattening);


end

== matlab function Simulator_Case_5/Control_PIDF_Discretized_And_Saturation/Anti_Wind-Up_Controller_And_Protection_Algorithm ==
  data: Heading_Error_Current input; Rudder_Angle_Command_Current output; Gain_Proportional input; Time_Integral input; Time_Derivative input; Time_Sampling input; Delta_Induced_Wind_Estimated input; Time_Current input
function Rudder_Angle_Command_Current = PIDF_Discretized_Anti_Wind_Up(Heading_Error_Current,...
                                                                      Gain_Proportional,...
                                                                      Time_Integral,...
                                                                      Time_Derivative,...
                                                                      Time_Sampling,...
                                                                      Delta_Induced_Wind_Estimated,...
                                                                      Time_Current)

% Anti Wind-Up online algorithm:
Rudder_Angle_Command_Current = PIDF_Discretized_Anti_Wind_Up_Saturation(Heading_Error_Current,...
                                                                        Gain_Proportional,...
                                                                        Time_Integral,...
                                                                        Time_Derivative,...
                                                                        Time_Sampling);

% % Persistents definition:
% persistent Heading_Error_Previous;
% persistent Heading_Error_Filtered_Previous;
% persistent Heading_Error_Filtered_Previous_Previous;
% persistent Rudder_Angle_Command_Previous;
% persistent Count_Persistent_Update;
% 
% % Threshold:
% Rudder_Angle_Minimal = -35*(pi/180);
% Rudder_Angle_Maximal = 35*(pi/180);
% 
% % Condition of persistent valorization:
% if isempty(Count_Persistent_Update)
%     Count_Persistent_Update = 0;
% end
% if isempty(Heading_Error_Previous)
%     Heading_Error_Previous = 0;
% end
% if isempty(Heading_Error_Filtered_Previous)
%     Heading_Error_Filtered_Previous = 0;
% end
% if isempty(Heading_Error_Filtered_Previous_Previous)
%     Heading_Error_Filtered_Previous_Previous = 0;
% end
% if isempty(Rudder_Angle_Command_Previous)
%     Rudder_Angle_Command_Previous = 0;
% end
% 
% % Calculate the current heading error filtered:
% Filter_Coefficient = 0.1;
% %Heading_Error_Filtered_Current = Heading_Error_Filtered_Previous*(1 - (Time_Sampling/(Filter_Coefficient*Time_Derivative))) + Heading_Error_Previous*(Time_Sampling/(Filter_Coefficient*Time_Derivative));
% Heading_Error_Filtered_Current = Heading_Error_Filtered_Previous*(1 - (Time_Sampling/(Filter_Coefficient*Time_Derivative))) + Heading_Error_Current*(Time_Sampling/(Filter_Coefficient*Time_Derivative));
% 
% % Define the increment of the command:
% Delta_Increment_Command_Current = Gain_Proportional*(Heading_Error_Current - Heading_Error_Previous) + ((Gain_Proportional*Time_Sampling)/Time_Integral)*Heading_Error_Current + ...
%                                   ((Gain_Proportional*Time_Derivative)/Time_Sampling)*(Heading_Error_Filtered_Current - 2*Heading_Error_Filtered_Previous + ...
%                                   Heading_Error_Filtered_Previous_Previous);
% % Delta_Increment_Command_Current = Gain_Proportional*(Heading_Error_Current - Heading_Error_Previous) + ((Gain_Proportional*Time_Sampling)/Time_Integral)*Heading_Error_Current + ...
% %                                   ((Gain_Proportional*Time_Derivative)/Time_Sampling)*(Heading_Error_Current - 2*Heading_Error_Previous + ...
% %                                   Heading_Error_Filtered_Previous_Previous);
% 
% % Update the output:
% % Anti wind-up condition:
% if ((Rudder_Angle_Command_Previous + Delta_Increment_Command_Current) > Rudder_Angle_Maximal) ||...
%         ((Rudder_Angle_Command_Previous + Delta_Increment_Command_Current) < Rudder_Angle_Minimal)
%     % Rudder_Angle_Command_Current = Rudder_Angle_Command_Previous;
%     % Use the estimator of the Wind uppon the action of the rudder:
%     % Rudder_Angle_Command_Current = Rudder_Angle_Command_Previous - Delta_Induced_Wind_Estimated;
%     Rudder_Angle_Command_Current = Rudder_Angle_Command_Previous;
% else
%     % Use the estimator of the Wind uppon the action of the rudder:
%     % Rudder_Angle_Command_Current = Rudder_Angle_Command_Previous + Delta_Increment_Command_Current;
%     Rudder_Angle_Command_Current = Rudder_Angle_Command_Previous + Delta_Increment_Command_Current - Delta_Induced_Wind_Estimated;
% end
% 
% % Update the persistents:
% Rudder_Angle_Command_Previous = Rudder_Angle_Command_Current;
% Heading_Error_Previous = Heading_Error_Current;
% Count_Persistent_Update = Count_Persistent_Update + 1;
% if Count_Persistent_Update == 1
%     Heading_Error_Filtered_Previous_Previous = 0;
% else
%     Heading_Error_Filtered_Previous_Previous = Heading_Error_Filtered_Previous;
% end
% Heading_Error_Filtered_Previous = Heading_Error_Filtered_Current;
% 
% % % Numerical protection for the error:
% % % if Heading_Error_Current > 2*pi || Heading_Error_Current < -2*pi
% % %     Rudder_Angle_Command_Current = Rudder_Angle_Command_Previous - Delta_Induced_Wind_Estimated;
% % % end
% % if isnan(Heading_Error_Current) 
% %     Rudder_Angle_Command_Current = Rudder_Angle_Command_Previous - Delta_Induced_Wind_Estimated;
% % end

end

== matlab function Simulator_Case_5/Environmental_Perturbations/Wind_Estimator ==
  data: Wind_Angle_Generated output; Wind_Velocity_Generated output; Wind_Speed output; Velocity_Ship input; Wind_Direction output; Table_Wind_Coefficients input; Yaw_Wind_Coefficient_Current output; Lenght_Ship_Overall input; Density_Air input; Area_Lateral_Projected_Wind input; Inertia_Ship_Vertical_Axis input; Heading_Induced_Wind output; Torque_Wind output; Time_Sampling input
function [Wind_Angle_Generated,...
          Wind_Velocity_Generated,...
          Wind_Speed,...
          Wind_Direction,...
          Yaw_Wind_Coefficient_Current,...
          Heading_Induced_Wind,...
          Torque_Wind] = Wind_Estimator(Velocity_Ship,...
                                        Table_Wind_Coefficients,...
                                        Lenght_Ship_Overall,...
                                        Density_Air,...
                                        Area_Lateral_Projected_Wind,...
                                        Inertia_Ship_Vertical_Axis,...
                                        Time_Sampling)

% Wind estimator and generator online algorithm:
[Wind_Angle_Generated,...
 Wind_Velocity_Generated,...
 Wind_Speed,...
 Wind_Direction,...
 Yaw_Wind_Coefficient_Current,...
 Heading_Induced_Wind,...
 Torque_Wind] = Wind_Estimator_Generator(Velocity_Ship,...
                                         Table_Wind_Coefficients,...
                                         Lenght_Ship_Overall,...
                                         Density_Air,...
                                         Area_Lateral_Projected_Wind,...
                                         Inertia_Ship_Vertical_Axis,...
                                         Time_Sampling);

end

== matlab function Simulator_Case_5/Navigation_And_Wave_Estimator/Wave_Identification_Parameters_ARMA ==
  data: Heading_Wave_High_Frequency_Estimated input; Wave_Pulsation_Estimated output; Wave_Damping_Factor_Estimated output; Time_Sampling input
function [Wave_Pulsation_Estimated,...
          Wave_Damping_Factor_Estimated] = Wave_Parameters_Identification_ARMA(Heading_Wave_High_Frequency_Estimated,...
                                                                               Time_Sampling)

% Two stage Recursive Extended least squares algorithm to estimate the wave
% pulsation and damping factor:
[Wave_Pulsation_Estimated,...
 Wave_Damping_Factor_Estimated] = Wave_Identification_ARMA(Heading_Wave_High_Frequency_Estimated,...
                                                           Time_Sampling);


end

== matlab function Simulator_Case_5/Navigation_And_Wave_Estimator/High_Pass_Filter ==
  data: Heading_Unfiltered_Input input; Heading_Filtered_Ouput output; Time_Sampling input
function Heading_Filtered_Ouput= High_Pass_Wave_Filter(Heading_Unfiltered_Input,...
                                                       Time_Sampling)

% Online numerical high-pass filter for pre-processing of the heading for
% identification:
Heading_Filtered_Ouput = High_Pass_Wave_Filter_Identification(Heading_Unfiltered_Input,...
                                                              Time_Sampling);

end

== matlab function Simulator_Case_5/Guidance_Heading/Guidance_Algorithm ==
  settings: updateMethod=DISCRETE
  data: Velocity_Current input; Heading_Aimed_Next output; Waypoints input; Position_X_Ship_Current input; Position_Y_Ship_Current input; Heading_Ship_Current input; Position_X_Final_Waypoint input; Position_Y_Final_Waypoint input; Time_Current input; Time_End_Guidance output
function [Heading_Aimed_Next,Time_End_Guidance] = Guidance_Waypoints_Following(Velocity_Current,...
                                                                               Waypoints,...
                                                                               Position_X_Ship_Current,...
                                                                               Position_Y_Ship_Current,...
                                                                               Heading_Ship_Current,...
                                                                               Position_X_Final_Waypoint,...
                                                                               Position_Y_Final_Waypoint,...
                                                                               Time_Current)

% Initialization:
if Time_Current == 0
    Position_X_Ship_Current = Waypoints(1,1);
    Position_Y_Ship_Current = Waypoints(1,2);
end

% Terminal point features:
Position_X_Final_Point = Position_X_Final_Waypoint;
Position_Y_Final_Point = Position_Y_Final_Waypoint;
Radius_Final_Waypoint = 50;

% Define persistent for heading protection:
persistent Heading_Previous;
if isempty(Heading_Previous)
    Heading_Previous = Heading_Ship_Current;
end

% Enable Guidance to work if the ship is not close to the final waypoint:
if ~((Position_X_Ship_Current - Position_X_Final_Point)^2 + (Position_Y_Ship_Current - Position_Y_Final_Point)^2 <= Radius_Final_Waypoint^2)

    % Then settle the time of end Guidance:
    Time_End_Guidance = 0;

    % Retreive the aimed heading angle that must be performed at this step time
    % of the simulation to follow the Waypoints generated trajectory:
    [Heading_Aimed_Unit,Heading_Aimed_Compass,...
     Heading_Error_Unit,Heading_Error_Compass,...
     Selected_Waypoints,Heading_Current_Unit] = Guidance_Heading_Rudder_Angle(Waypoints,...
                                                                              Position_X_Ship_Current,...
                                                                              Position_Y_Ship_Current, ...
                                                                              Heading_Ship_Current);

    % Update the heading aimed:
    Heading_Aimed_Next = Heading_Aimed_Compass;

    % Then update the persistent:
    Heading_Previous = Heading_Aimed_Next;       

else
    
    [Heading_Aimed_Unit,Heading_Aimed_Compass,...
     Heading_Error_Unit,Heading_Error_Compass,...
     Selected_Waypoints,Heading_Current_Unit] = Guidance_Heading_Rudder_Angle(Waypoints,...
                                                                              Position_X_Ship_Current,...
                                                                              Position_Y_Ship_Current, ...
                                                                              Heading_Ship_Current);

    % Update the heading aimed:
    Heading_Aimed_Next = Heading_Aimed_Compass;

    % Then update the persistent:
    Heading_Previous = Heading_Aimed_Next; 
    
    % Then determine the end time of the Guidance scheme:
    Time_End_Guidance = Time_Current;

end
end

== matlab function Simulator_Case_5/Navigation_And_Wave_Estimator/Sensors_Fusion_And_Filtering/Real_Navigation_Sensors/Conversion_ENU_To_LLA_Coordinates ==
  data: Altitude_Current output; Latitude_Current output; Longitude_Current output; Component_X_ENU input; Component_Y_ENU input; Component_Z_ENU input
function [Altitude_Current,Latitude_Current,Longitude_Current] = Conversion_ENU_To_LAA(Component_X_ENU,...
                                                                                       Component_Y_ENU,...
                                                                                       Component_Z_ENU)

% This function serves as a mean to convert ENU coordinates into LLA
% coordinates. Need to write an embedded function to be injected in the
% Mission Software.
% Reference point for the current mission;
Reference_Point_Port_Mahon = [43.059023,3.002915,0];
Position_Vector_ENU_Current = [Component_X_ENU,Component_Y_ENU,Component_Z_ENU];

% Conversion using Matlab function:
Position_Vector_LLA_Current = enu2lla(Position_Vector_ENU_Current,Reference_Point_Port_Mahon,'ellipsoid');

% Feed the outputs:
Latitude_Current = Position_Vector_LLA_Current(1);
Altitude_Current = Position_Vector_LLA_Current(3);
Longitude_Current = Position_Vector_LLA_Current(2);

end

== matlab function Simulator_Case_5/Navigation_And_Wave_Estimator/Sensors_Fusion_And_Filtering/Kinematics_Propagator_GPS ==
  settings: updateMethod=DISCRETE
  data: Velocity_Current input; Heading_Angle_Current_Mes input; Position_X_Ship_Init input; Position_Y_Ship_Init input; Time_Simulation_Current input; Position_X_Ship_Compass_Next output; Position_Y_Ship_Compass_Next output; Acceleration_X_Ship_Next output; Acceleration_Y_Ship_Next output; Velocity_X_Ship_Next_Local output; Velocity_Y_Ship_Next_Local output; Time_Sampling input
function [Position_X_Ship_Compass_Next,...
          Position_Y_Ship_Compass_Next,...
          Acceleration_X_Ship_Next,...
          Acceleration_Y_Ship_Next,...
          Velocity_X_Ship_Next_Local,...
          Velocity_Y_Ship_Next_Local] = Kinematics_Propagation(Velocity_Current,...
                                                               Heading_Angle_Current_Mes,...
                                                               Position_X_Ship_Init,...
                                                               Position_Y_Ship_Init,...
                                                               Time_Simulation_Current,...
                                                               Time_Sampling)

% Persistents definition:
persistent Position_X_Ship_Compass_Prev
persistent Position_Y_Ship_Compass_Prev
persistent Heading_Previous
persistent Velocity_X_Ship_Local_Previous
persistent Velocity_Y_Ship_Local_Previous

% Heading previous storage:
if isempty(Heading_Previous)
    Heading_Previous = Heading_Angle_Current_Mes;
    Heading_Current = Heading_Previous;
else
    Heading_Current = Heading_Angle_Current_Mes;
end

% Calculate the local position increment but use both convention (unit and compass):
% Compass:
Position_X_Ship_Current_Increment_Compass = Time_Sampling*Velocity_Current*sin(Heading_Previous);
Position_Y_Ship_Current_Increment_Compass = Time_Sampling*Velocity_Current*cos(Heading_Previous);

% The simple velocity discrete increment:
Velocity_X_Ship_Local = Velocity_Current*sin(Heading_Angle_Current_Mes);
Velocity_Y_Ship_Local = Velocity_Current*cos(Heading_Angle_Current_Mes);

if isempty(Velocity_X_Ship_Local_Previous)
    Velocity_X_Ship_Local_Previous = Velocity_Current*sin(Heading_Angle_Current_Mes);
    Acceleration_X_Ship_Next = 0;
else
    Acceleration_X_Ship_Next = (Velocity_X_Ship_Local - Velocity_X_Ship_Local_Previous)/Time_Sampling;
    Velocity_X_Ship_Local_Previous = Velocity_X_Ship_Local;
end
if isempty(Velocity_Y_Ship_Local_Previous)
    Velocity_Y_Ship_Local_Previous = Velocity_Current*cos(Heading_Angle_Current_Mes);
    Acceleration_Y_Ship_Next = 0;
else
    Acceleration_Y_Ship_Next = (Velocity_Y_Ship_Local - Velocity_Y_Ship_Local_Previous)/Time_Sampling;
    Velocity_Y_Ship_Local_Previous = Velocity_Y_Ship_Local;
end


% Compass position persistent filling:
if isempty(Position_X_Ship_Compass_Prev)
    Position_X_Ship_Compass_Prev = Position_X_Ship_Init + Position_X_Ship_Current_Increment_Compass;
else
    Position_X_Ship_Compass_Prev = Position_X_Ship_Compass_Prev + Position_X_Ship_Current_Increment_Compass;
end
if isempty(Position_Y_Ship_Compass_Prev)
    Position_Y_Ship_Compass_Prev = Position_Y_Ship_Init + Position_Y_Ship_Current_Increment_Compass;
else
    Position_Y_Ship_Compass_Prev = Position_Y_Ship_Compass_Prev + Position_Y_Ship_Current_Increment_Compass;
end

% Then update the outputs:
% Compass:
Position_X_Ship_Compass_Next = Position_X_Ship_Compass_Prev;
Position_Y_Ship_Compass_Next = Position_Y_Ship_Compass_Prev;

% Store the heading:
Heading_Estimated_Next = Heading_Current;
Heading_Previous = Heading_Estimated_Next;

% Velocity:
Velocity_X_Ship_Next_Local = Velocity_X_Ship_Local;
Velocity_Y_Ship_Next_Local = Velocity_Y_Ship_Local;

end

== matlab function Simulator_Case_5/Navigation_And_Wave_Estimator/Wave_Estimation_Kalman_Filter/Wave_Heading_Estimation ==
  data: Heading_Total_Observed_Current input; Rudder_Angle_Commanded_Current input; Wave_Pulsation_Estimated input; Damping_Wave_Estimated input; Time_Current input; Time_Constant_Ship input; Gain_Ship input; Time_Sampling input; Noise_For_Heading_wave input; Heading_Rate_Wave_Estimated_Current output; Heading_Wave_Estimated_Current output; Heading_Low_Frequency_Estimated_Current output; Heading_Rate_Estimated_Current output; Bias_Estimated_Current output; Covariance_Aposteriori_Estimate output; Torque_Wind_Estimated_Input input; Inertia_Ship_Vertical input; Wave_Pulsation_Identified input
function [Heading_Rate_Wave_Estimated_Current,...
          Heading_Wave_Estimated_Current,...
          Heading_Low_Frequency_Estimated_Current,...
          Heading_Rate_Estimated_Current,...
          Bias_Estimated_Current,...
          Covariance_Aposteriori_Estimate]= Kalman_Filter_Wave_Estimation(Heading_Total_Observed_Current,...
                                                                          Rudder_Angle_Commanded_Current,...
                                                                          Wave_Pulsation_Estimated,...
                                                                          Damping_Wave_Estimated,...
                                                                          Time_Current,...
                                                                          Time_Constant_Ship,...
                                                                          Gain_Ship,...
                                                                          Time_Sampling,...
                                                                          Noise_For_Heading_wave,...
                                                                          Torque_Wind_Estimated_Input,...
                                                                          Inertia_Ship_Vertical,...
                                                                          Wave_Pulsation_Identified)

% Online Wave Observer Kalman algorithm for better wave high frequency
% filtering:
[Heading_Rate_Wave_Estimated_Current,...
 Heading_Wave_Estimated_Current,...
 Heading_Low_Frequency_Estimated_Current,...
 Heading_Rate_Estimated_Current,...
 Bias_Estimated_Current,...
 Covariance_Aposteriori_Estimate] = Kalman_Observer_Wave_Estimation(Heading_Total_Observed_Current,...
                                                                    Rudder_Angle_Commanded_Current,...
                                                                    Wave_Pulsation_Estimated,...
                                                                    Damping_Wave_Estimated,...
                                                                    Time_Current,...
                                                                    Time_Constant_Ship,...
                                                                    Gain_Ship,...
                                                                    Time_Sampling,...
                                                                    Noise_For_Heading_wave,...
                                                                    Torque_Wind_Estimated_Input,...
                                                                    Inertia_Ship_Vertical,...
                                                                    Wave_Pulsation_Identified);

end
